simulink model "Sim_Ex16"  (R2017a)
settings: Solver=VariableStepAuto  StartTime=0.0  StopTime=Stop_Time  MaxStep=1e-4  RelTol=1e-3
values from neighbouring files (symbols this model uses):
  Idqsr_Ref_Set = [0 -5;0 10]    [A_Ex16.m]
  Ki_Mat = Wcc*(Rs_Hat+Ra)*eye(2)    [A_Ex16.m]
  Kp_Mat = Wcc*[Lds_Hat 0;0 Lqs_Hat]    [A_Ex16.m]
  Lamf = 0.254    [A_Ex16.m]
  Lamf_Hat = 1.0*Lamf    (= 0.254)    [A_Ex16.m]
  Lds = 3.6e-3    (= 0.0036)    [A_Ex16.m]
  Lqs = 4.3e-3    (= 0.0043)    [A_Ex16.m]
  p = 3    [A_Ex16.m]
  Ra = 10*Rs_Hat    (= 1.5)    [A_Ex16.m]
  Rs = 0.15    [A_Ex16.m]
  Step_Time = 0.005    [A_Ex16.m]
  Stop_Time = 0.1    [A_Ex16.m]
  Thetarm_Init = 0*pi*1/p    (= 0)    [A_Ex16.m]
  Wrm_Fin = 4000*2*pi/60    (= 418.879020479)    [A_Ex16.m]
  Wrm_Init = 4000*2*pi/60    (= 418.879020479)    [A_Ex16.m]
libraries: simulink x1
settings Model: Creator=KYC  LastModifiedBy=KYC

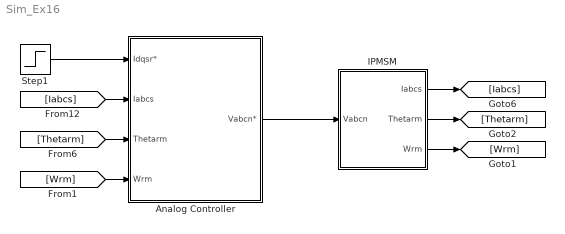
== system Sim_Ex16 ==
  Analog Controller : Subsystem
  IPMSM : Subsystem
  Step1 : Step  Time=Step_Time  Before=Idqsr_Ref_Set(:,1)  After=Idqsr_Ref_Set(:,2)
  wires:
  Analog Controller/1(Vabcn*) -> IPMSM/1(Vabcn)
  [Iabcs] -> Analog Controller/2(Iabcs)
  [Thetarm] -> Analog Controller/3(Thetarm)
  IPMSM/2(Thetarm) -> [Thetarm]
  IPMSM/1(Iabcs) -> [Iabcs]
  Step1/1 -> Analog Controller/1(Idqsr*)
  IPMSM/3(Wrm) -> [Wrm]
  [Wrm] -> Analog Controller/4(Wrm)

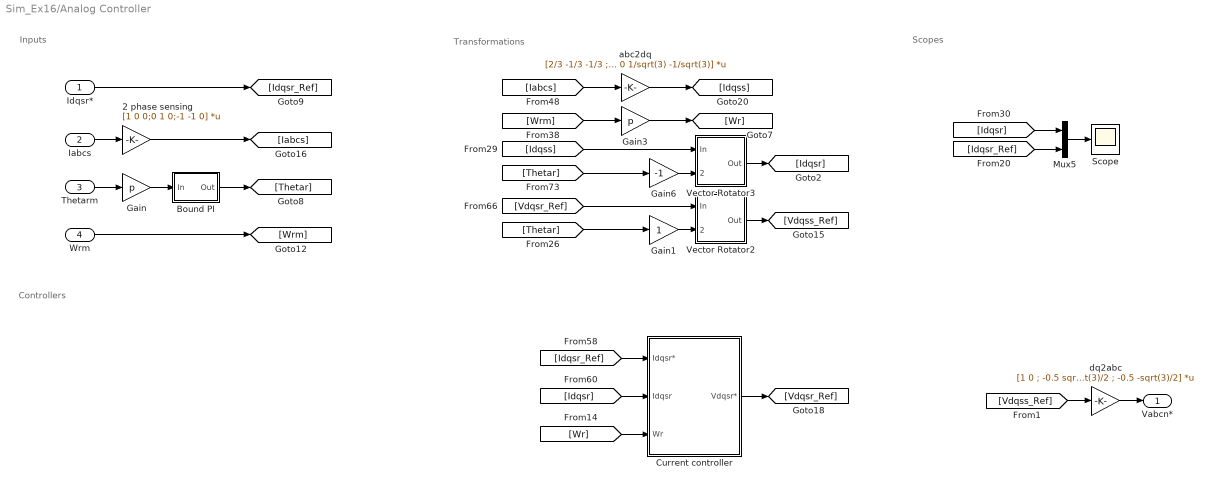
== system Sim_Ex16/Analog Controller ==
  note: Controllers
  note: Inputs
  note: Transformations
  note: Scopes
  Idqsr* : Inport
  Iabcs : Inport  Port=2
  Thetarm : Inport  Port=3
  Wrm : Inport  Port=4
  2 phase sensing : Gain  Gain=[1 0 0;0 1 0;-1 -1 0]  Multiplication=Matrix(K*u)  SaturateOnIntegerOverflow=on  OutDataTypeStr=Inherit: Same as input  ParamDataTypeStr=Inherit: Same as input
  Bound PI : Subsystem
  Current controller : Subsystem
  Gain : Gain  Gain=p
  Gain1 : Gain
  Gain3 : Gain  Gain=p
  Gain6 : Gain  Gain=-1
  Mux5 : Mux  Inputs=2
  Scope : Scope
  Vector Rotator2 : Subsystem
  Vector Rotator3 : Subsystem
  abc2dq : Gain  Gain=[2/3 -1/3 -1/3 ; 0 1/sqrt(3) -1/sqrt(3)]  Multiplication=Matrix(K*u)  SaturateOnIntegerOverflow=on  OutDataTypeStr=Inherit: Same as input  ParamDataTypeStr=Inherit: Same as input
  dq2abc : Gain  Gain=[1 0 ; -0.5 sqrt(3)/2 ; -0.5 -sqrt(3)/2]  Multiplication=Matrix(K*u)
  Vabcn* : Outport  InitialOutput=[0]
  wires:
  [Idqsr] -> Current controller/2(Idqsr)
  [Idqsr_Ref] -> Current controller/1(Idqsr*)
  Thetarm/1 -> Gain/1
  [Wr] -> Current controller/3(Wr)
  Gain/1 -> Bound PI/1(In)
  Bound PI/1(Out) -> [Thetar]
  Current controller/1(Vdqsr*) -> [Vdqsr_Ref]
  dq2abc/1 -> Vabcn*/1
  [Thetar] -> Gain1/1
  [Vdqsr_Ref] -> Vector Rotator2/1(In)
  Vector Rotator2/1(Out) -> [Vdqss_Ref]
  Gain6/1 -> Vector Rotator3/2(Theta)
  [Idqss] -> Vector Rotator3/1(In)
  Vector Rotator3/1(Out) -> [Idqsr]
  [Thetar] -> Gain6/1
  Iabcs/1 -> 2 phase sensing/1
  2 phase sensing/1 -> [Iabcs]
  Wrm/1 -> [Wrm]
  Idqsr*/1 -> [Idqsr_Ref]
  [Idqsr] -> Mux5/1
  [Idqsr_Ref] -> Mux5/2
  [Vdqss_Ref] -> dq2abc/1
  Mux5/1 -> Scope/1
  Gain1/1 -> Vector Rotator2/2(Theta)
  [Wrm] -> Gain3/1
  Gain3/1 -> [Wr]
  [Iabcs] -> abc2dq/1
  abc2dq/1 -> [Idqss]

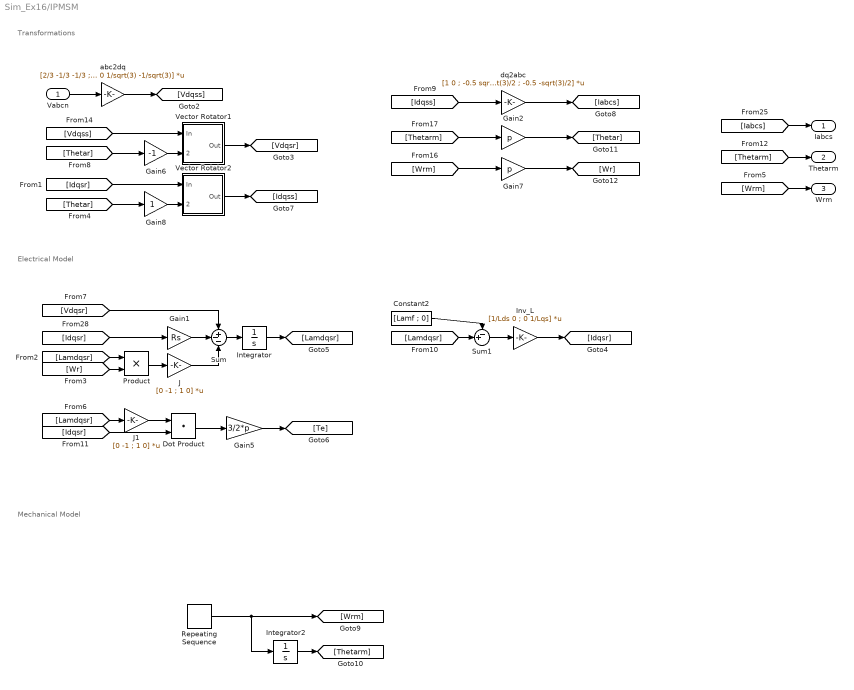
== system Sim_Ex16/IPMSM ==
  note: Transformations
  note: Electrical Model
  note: Mechanical Model
  Vabcn : Inport
  Constant2 : Constant  Value=[Lamf ; 0]
  Dot Product : DotProduct  InputSameDT=on  OutDataTypeStr=Inherit: Inherit via internal rule
  Gain1 : Gain  Gain=Rs
  Gain2 : Gain  Gain=p
  Gain5 : Gain  Gain=3/2*p
  Gain6 : Gain  Gain=-1
  Gain7 : Gain  Gain=p
  Gain8 : Gain
  Integrator : Integrator  InitialCondition=[Lamf ; 0]
  Integrator2 : Integrator  InitialCondition=Thetarm_Init  WrapState=on
  Inv_L : Gain  Gain=[1/Lds 0 ; 0 1/Lqs]  Multiplication=Matrix(K*u)
  J : Gain  Gain=[0 -1 ; 1 0]  Multiplication=Matrix(K*u)
  J1 : Gain  Gain=[0 -1 ; 1 0]  Multiplication=Matrix(K*u)
  Product : Product  RndMeth=Zero
  Repeating Sequence : simulink/Sources/Repeating Sequence  rep_seq_t=[0 Stop_Time]  rep_seq_y=[Wrm_Init Wrm_Fin]
  Sum : Sum  Inputs=+--
  Sum1 : Sum  Inputs=-+|
  Vector Rotator1 : Subsystem
  Vector Rotator2 : Subsystem
  abc2dq : Gain  Gain=[2/3 -1/3 -1/3 ; 0 1/sqrt(3) -1/sqrt(3)]  Multiplication=Matrix(K*u)  SaturateOnIntegerOverflow=on  OutDataTypeStr=Inherit: Same as input  ParamDataTypeStr=Inherit: Same as input
  dq2abc : Gain  Gain=[1 0 ; -0.5 sqrt(3)/2 ; -0.5 -sqrt(3)/2]  Multiplication=Matrix(K*u)
  Iabcs : Outport
  Thetarm : Outport  Port=2
  Wrm : Outport  Port=3
  wires:
  [Iabcs] -> Iabcs/1
  [Wrm] -> Gain7/1
  [Thetarm] -> Gain2/1
  Gain7/1 -> [Wr]
  dq2abc/1 -> [Iabcs]
  [Idqss] -> dq2abc/1
  Vector Rotator2/1(Out) -> [Idqss]
  [Idqsr] -> Vector Rotator2/1(In)
  Vector Rotator1/1(Out) -> [Vdqsr]
  [Thetarm] -> Thetarm/1
  Gain2/1 -> [Thetar]
  [Thetar] -> Gain6/1
  Gain6/1 -> Vector Rotator1/2(Theta)
  [Thetar] -> Gain8/1
  Gain8/1 -> Vector Rotator2/2(Theta)
  Integrator2/1 -> [Thetarm]
  Repeating Sequence/1 -> [Wrm], Integrator2/1
  Sum1/1 -> Inv_L/1
  Inv_L/1 -> [Idqsr]
  [Lamdqsr] -> Sum1/2
  Constant2/1 -> Sum1/1
  Dot Product/1 -> Gain5/1
  J1/1 -> Dot Product/1
  [Lamdqsr] -> J1/1
  [Idqsr] -> Dot Product/2
  Gain5/1 -> [Te]
  Integrator/1 -> [Lamdqsr]
  [Vdqsr] -> Sum/1
  [Lamdqsr] -> Product/1
  Sum/1 -> Integrator/1
  [Wr] -> Product/2
  Product/1 -> J/1
  [Idqsr] -> Gain1/1
  J/1 -> Sum/3
  Gain1/1 -> Sum/2
  Vabcn/1 -> abc2dq/1
  abc2dq/1 -> [Vdqss]
  [Vdqss] -> Vector Rotator1/1(In)
  [Wrm] -> Wrm/1

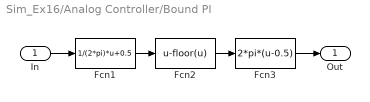
== system Sim_Ex16/Analog Controller/Bound PI ==
  In : Inport
  Fcn1 : Fcn  Expr=1/(2*pi)*u+0.5
  Fcn2 : Fcn  Expr=u-floor(u)
  Fcn3 : Fcn  Expr=2*pi*(u-0.5)
  Out : Outport
  wires:
  Fcn1/1 -> Fcn2/1
  Fcn2/1 -> Fcn3/1
  In/1 -> Fcn1/1
  Fcn3/1 -> Out/1

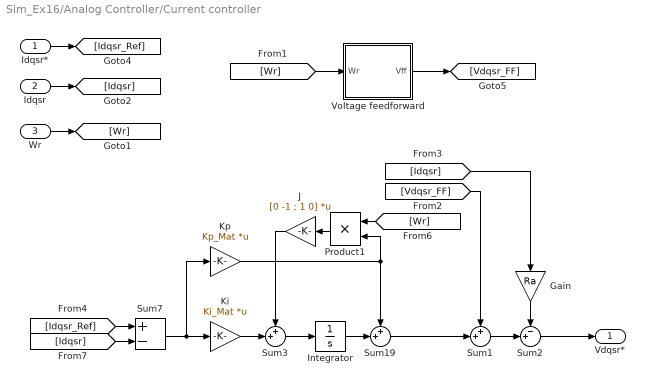
== system Sim_Ex16/Analog Controller/Current controller ==
  Idqsr* : Inport
  Idqsr : Inport  Port=2
  Wr : Inport  Port=3
  Gain : Gain  Gain=Ra
  Integrator : Integrator
  J : Gain  Gain=[0 -1 ; 1 0]  Multiplication=Matrix(K*u)
  Ki : Gain  Gain=Ki_Mat  Multiplication=Matrix(K*u)  SaturateOnIntegerOverflow=on  OutDataTypeStr=Inherit: Same as input  ParamDataTypeStr=Inherit: Same as input
  Kp : Gain  Gain=Kp_Mat  Multiplication=Matrix(K*u)  SaturateOnIntegerOverflow=on  OutDataTypeStr=Inherit: Same as input  ParamDataTypeStr=Inherit: Same as input
  Product1 : Product  RndMeth=Zero
  Sum1 : Sum  Inputs=++|
  Sum19 : Sum  Inputs=++|
  Sum2 : Sum  Inputs=-+|
  Sum3 : Sum  Inputs=++|
  Sum7 : Sum  Inputs=+-
  Voltage feedforward : Subsystem
  Vdqsr* : Outport
  wires:
  [Vdqsr_FF] -> Sum1/1
  Integrator/1 -> Sum19/2
  Sum7/1 -> Kp/1, Ki/1
  Idqsr/1 -> [Idqsr]
  Kp/1 -> Product1/2, Sum19/1
  Idqsr*/1 -> [Idqsr_Ref]
  [Idqsr_Ref] -> Sum7/1
  [Idqsr] -> Sum7/2
  Wr/1 -> [Wr]
  [Wr] -> Voltage feedforward/1(Wr)
  Voltage feedforward/1(Vff) -> [Vdqsr_FF]
  Sum1/1 -> Sum2/2
  Sum2/1 -> Vdqsr*/1
  Gain/1 -> Sum2/1
  [Idqsr] -> Gain/1
  [Wr] -> Product1/1
  Sum3/1 -> Integrator/1
  Ki/1 -> Sum3/2
  J/1 -> Sum3/1
  Sum19/1 -> Sum1/2
  Product1/1 -> J/1

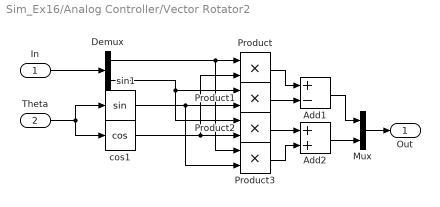
== system Sim_Ex16/Analog Controller/Vector Rotator2 ==
  In : Inport
  Theta : Inport  Port=2
  Add1 : Sum  Inputs=+-
  Add2 : Sum
  Demux : Demux  Outputs=2
  Mux : Mux  Inputs=[1 1]
  Product{,1..3} (4 alike) : Product  RndMeth=Zero
  cos1 : Trigonometry  Operator=cos
  sin1 : Trigonometry
  Out : Outport
  wires:
  Theta/1 -> cos1/1, sin1/1
  Demux/1 -> Product3/1, Product/1
  Mux/1 -> Out/1
  In/1 -> Demux/1
  Demux/2 -> Product1/1, Product2/1
  cos1/1 -> Product/2, Product2/2
  sin1/1 -> Product1/2, Product3/2
  Product/1 -> Add1/1
  Product1/1 -> Add1/2
  Add1/1 -> Mux/1
  Product2/1 -> Add2/1
  Product3/1 -> Add2/2
  Add2/1 -> Mux/2

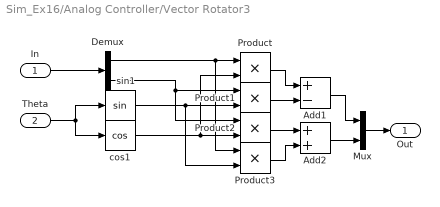
== system Sim_Ex16/Analog Controller/Vector Rotator3 ==
  In : Inport
  Theta : Inport  Port=2
  Add1 : Sum  Inputs=+-
  Add2 : Sum
  Demux : Demux  Outputs=2
  Mux : Mux  Inputs=[1 1]
  Product{,1..3} (4 alike) : Product  RndMeth=Zero
  cos1 : Trigonometry  Operator=cos
  sin1 : Trigonometry
  Out : Outport
  wires:
  Theta/1 -> cos1/1, sin1/1
  Demux/1 -> Product3/1, Product/1
  Mux/1 -> Out/1
  In/1 -> Demux/1
  Demux/2 -> Product1/1, Product2/1
  cos1/1 -> Product/2, Product2/2
  sin1/1 -> Product1/2, Product3/2
  Product/1 -> Add1/1
  Product1/1 -> Add1/2
  Add1/1 -> Mux/1
  Product2/1 -> Add2/1
  Product3/1 -> Add2/2
  Add2/1 -> Mux/2

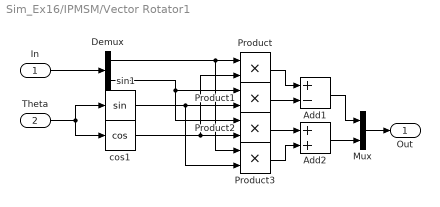
== system Sim_Ex16/IPMSM/Vector Rotator1 ==
  In : Inport
  Theta : Inport  Port=2
  Add1 : Sum  Inputs=+-
  Add2 : Sum
  Demux : Demux  Outputs=2
  Mux : Mux  Inputs=[1 1]
  Product{,1..3} (4 alike) : Product  RndMeth=Zero
  cos1 : Trigonometry  Operator=cos
  sin1 : Trigonometry
  Out : Outport
  wires:
  Add2/1 -> Mux/2
  Product3/1 -> Add2/2
  Product2/1 -> Add2/1
  Add1/1 -> Mux/1
  Product1/1 -> Add1/2
  Product/1 -> Add1/1
  sin1/1 -> Product3/2, Product1/2
  cos1/1 -> Product2/2, Product/2
  Demux/2 -> Product2/1, Product1/1
  In/1 -> Demux/1
  Mux/1 -> Out/1
  Demux/1 -> Product/1, Product3/1
  Theta/1 -> sin1/1, cos1/1

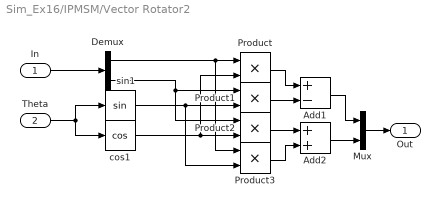
== system Sim_Ex16/IPMSM/Vector Rotator2 ==
  In : Inport
  Theta : Inport  Port=2
  Add1 : Sum  Inputs=+-
  Add2 : Sum
  Demux : Demux  Outputs=2
  Mux : Mux  Inputs=[1 1]
  Product{,1..3} (4 alike) : Product  RndMeth=Zero
  cos1 : Trigonometry  Operator=cos
  sin1 : Trigonometry
  Out : Outport
  wires:
  Theta/1 -> cos1/1, sin1/1
  Demux/1 -> Product3/1, Product/1
  Mux/1 -> Out/1
  In/1 -> Demux/1
  Demux/2 -> Product1/1, Product2/1
  cos1/1 -> Product/2, Product2/2
  sin1/1 -> Product1/2, Product3/2
  Product/1 -> Add1/1
  Product1/1 -> Add1/2
  Add1/1 -> Mux/1
  Product2/1 -> Add2/1
  Product3/1 -> Add2/2
  Add2/1 -> Mux/2

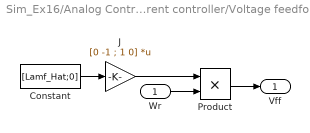
== system Sim_Ex16/Analog Controller/Current controller/Voltage feedforward ==
  Wr : Inport
  Constant : Constant  Value=[Lamf_Hat;0]
  J : Gain  Gain=[0 -1 ; 1 0]  Multiplication=Matrix(K*u)
  Product : Product  RndMeth=Zero
  Vff : Outport
  wires:
  Wr/1 -> Product/2
  J/1 -> Product/1
  Product/1 -> Vff/1
  Constant/1 -> J/1
